simulink model "Vicon_server_multi_robot_test_3_robots"  (R2022b)
settings: Solver=ode2  StartTime=0.0  StopTime=inf  FixedStep=0.001  RelTol=1e-3  EnableMultiTasking=on
InitFcn:
  | %set_param('MS_FR/MISSION SERVER QDRONE POSITION CONTROL/Trajectory Enable', 'sw', '0' )
  | %set_param('MS_FR/MISSION SERVER QDRONE POSITION CONTROL/Command Enable', 'sw', '0' )
undefined symbols (not defined in the file or in its folder): qc_get_step_size
libraries: quarc_library x10, simulink x3
settings Model: SimulationMode=external  ExtModeTrigDuration=10000  Creator=Admin  LastModifiedBy=user
settings SolverCC: AlgebraicLoopSolver=TrustRegion  PositivePriorityOrder=on  AutoInsertRateTranBlk=on
settings DataIOCC: ReturnWorkspaceOutputs=off
settings DebuggingCC: UnconnectedInputMsg=warning  UnconnectedOutputMsg=warning  UnconnectedLineMsg=warning  SFUnexpectedBacktrackingDiag=warning  SFNoUnconditionalDefaultTransitionDiag=warning  SFExecutionAtInitializationDiag=none  SFMachineParentedDataDiag=warning  ArithmeticOperatorsInVariantConditions=warning
settings ModelReferenceCC: EnableRefExpFcnMdlSchedulingChecks=on
settings SFSimCC: SimUseLocalCustomCode=off  CustomCodeUndefinedFunction=UseInterfaceOnly
settings RTWCC: Description=QUARC Win64 Target Using Toolchain  SystemTargetFile=quarc_win64.tlc  TemplateMakefile=quarc_default_tmf  RTWUseLocalCustomCode=off  Toolchain=QUARC win64 | nmake (64-bit Windows)  BuildConfiguration=Faster Runs
settings CodeAppCC: StateflowObjectComments=on
settings STFCustomTargetCC: ConcurrentExecutionCompliant=on  GRTInterface=on  UseToolchainInfoCompliant=on  SystemTargetFile=quarc_win64.tlc
settings GRTTargetCC: TargetLangStandard=C89/C90 (ANSI)  ParMdlRefBuildCompliant=off  CompOptLevelCompliant=off  CombineOutputUpdateFcns=off  MatFileLogging=off  CPPClassGenCompliant=off  GRTInterface=on  ExtMode=on  ExtModeMexFile=quarc_comm  ExtModeMexArgs='-w -d %d -uri %u', 'tcpip://192.168.0.5:17005'
settings ConfigComp: CovMetricSettings=dw  CovSaveCumulativeToWorkspaceVar=on  CovSaveSingleToWorkspaceVar=on  CovExternalEMLEnable=off

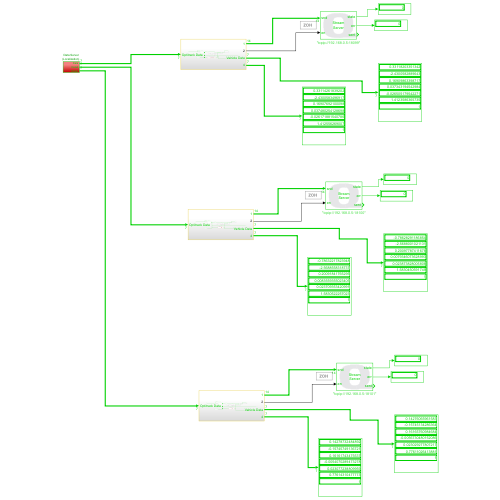
[thumbnail: Simulink's stored preview of the top-level diagram]
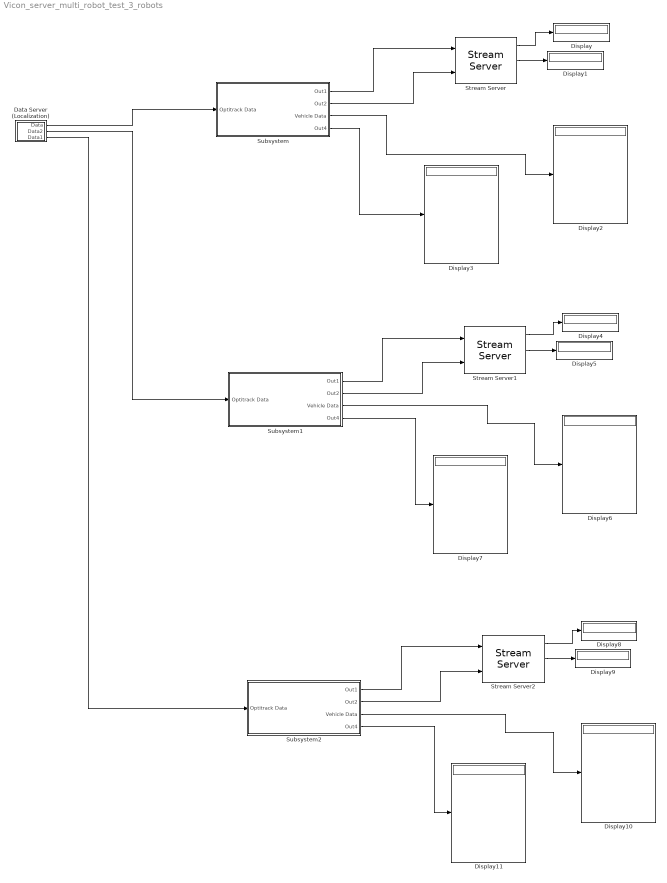
== system Vicon_server_multi_robot_test_3_robots ==
  "Data Server (Localization) " : Subsystem
  Display{,1..11} (12 alike) : Display
  Stream Server : quarc_library/Communications/Basic/Stream Server  uri_source=Specify via dialog (do not evaluate)  uri=tcpip://192.168.0.5:18099  send_buffer_size=1460  receive_buffer_size=1460  byte_order=little endian (Intel - LSB first)  optimization=Minimum latency  send_options=Send most recent data  receive_options=Do not receive data  default_value=[0]  sample_time=qc_get_step_size*2  active=off  implementation=Use blocking I/O in a separate thread  send_fifo_size=1000  receive_fifo_size=1000  send_priority=0  receive_priority=0  send_dimensions=off  receive_dimensions=off  max_dimensions=-1  data_type=Inherited via back propagation  type_expr=BusObject
      settings: AttributesFormatString="\"tcpip://192.168.0.5:18099\""
  Stream Server1 : quarc_library/Communications/Basic/Stream Server  uri_source=Specify via dialog (do not evaluate)  uri=tcpip://192.168.0.5:18100  send_buffer_size=1460  receive_buffer_size=1460  byte_order=little endian (Intel - LSB first)  optimization=Minimum latency  send_options=Send most recent data  receive_options=Do not receive data  default_value=[0]  sample_time=qc_get_step_size*2  active=off  implementation=Use blocking I/O in a separate thread  send_fifo_size=1000  receive_fifo_size=1000  send_priority=0  receive_priority=0  send_dimensions=off  receive_dimensions=off  max_dimensions=-1  data_type=Inherited via back propagation  type_expr=BusObject
      settings: AttributesFormatString="\"tcpip://192.168.0.5:18100\""
  Stream Server2 : quarc_library/Communications/Basic/Stream Server  uri_source=Specify via dialog (do not evaluate)  uri=tcpip://192.168.0.5:18101  send_buffer_size=1460  receive_buffer_size=1460  byte_order=little endian (Intel - LSB first)  optimization=Minimum latency  send_options=Send most recent data  receive_options=Do not receive data  default_value=[0]  sample_time=qc_get_step_size*2  active=off  implementation=Use blocking I/O in a separate thread  send_fifo_size=1000  receive_fifo_size=1000  send_priority=0  receive_priority=0  send_dimensions=off  receive_dimensions=off  max_dimensions=-1  data_type=Inherited via back propagation  type_expr=BusObject
      settings: AttributesFormatString="\"tcpip://192.168.0.5:18101\""
  Subsystem : Subsystem
  Subsystem1 : Subsystem
  Subsystem2 : Subsystem
  wires:
  Stream Server/1 -> Display/1
  Stream Server/2 -> Display1/1
  Subsystem/1(Out1) -> Stream Server/1
  Subsystem/2(Out2) -> Stream Server/2
  Subsystem/3(Vehicle Data) -> Display2/1
  Subsystem/4(Out4) -> Display3/1
  Stream Server1/1 -> Display4/1
  Stream Server1/2 -> Display5/1
  Subsystem1/4(Out4) -> Display7/1
  Subsystem1/1(Out1) -> Stream Server1/1
  Subsystem1/2(Out2) -> Stream Server1/2
  Subsystem1/3(Vehicle Data) -> Display6/1
  "Data Server (Localization) "/1(Data) -> Subsystem/1(Optitrack Data)
  "Data Server (Localization) "/2(Data2) -> Subsystem1/1(Optitrack Data)
  Subsystem2/2(Out2) -> Stream Server2/2
  Subsystem2/3(Vehicle Data) -> Display10/1
  Stream Server2/2 -> Display9/1
  Subsystem2/4(Out4) -> Display11/1
  Stream Server2/1 -> Display8/1
  Subsystem2/1(Out1) -> Stream Server2/1
  "Data Server (Localization) "/3(Data1) -> Subsystem2/1(Optitrack Data)

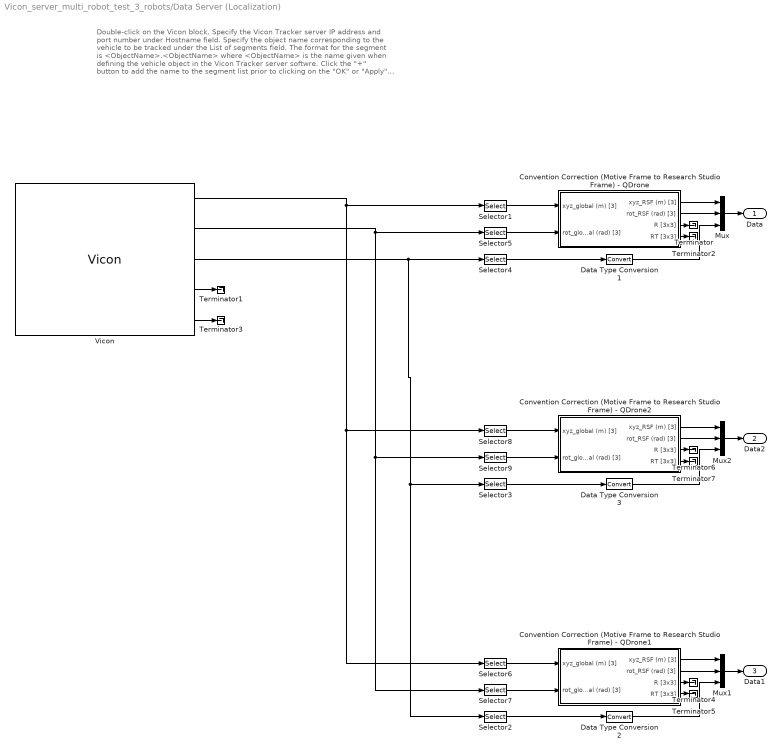
== system Vicon_server_multi_robot_test_3_robots/Data Server (Localization)  ==
  note: Double-click on the Vicon block.
      |
      | Specify the Vicon Tracker server IP address and port number under Hostname field.
      |
      | Specify the object name corresponding to the vehicle to be tracked under the
      | List of segments field. The format for the segment is <ObjectName>.<ObjectName>
      | where <ObjectName> is the name given when defining the vehicle object in the
      | Vicon Tracker server softwre. Click the "+" button to add the name to the segment list
      | prior to clicking on the "OK" or "Apply" button.
      | Remove extra/unused entries from the list using the "-" button.
      |
      | Make sure the checkbox next to the Object name inside the Object tab
      | in Vicon Tracker software is selected/checked and Tracker is streaming (Live) tracking
      | data before running this model.
  Convention Correction (Motive Frame to Research Studio Frame) - QDrone : Subsystem
  Convention Correction (Motive Frame to Research Studio Frame) - QDrone1 : Subsystem
  Convention Correction (Motive Frame to Research Studio Frame) - QDrone2 : Subsystem
  Data Type Conversion1 : DataTypeConversion  SaturateOnIntegerOverflow=off  RndMeth=Floor
  Data Type Conversion2 : DataTypeConversion  SaturateOnIntegerOverflow=off  RndMeth=Floor
  Data Type Conversion3 : DataTypeConversion  SaturateOnIntegerOverflow=off  RndMeth=Floor
  Mux : Mux  Inputs=3
  Mux1 : Mux  Inputs=3
  Mux2 : Mux  Inputs=3
  Selector1 : Selector  InputPortWidth=9  IndexOptions=Index vector (dialog)  Indices=[1:3]  OutputSizes=1
  Selector2 : Selector  InputPortWidth=3  IndexOptions=Index vector (dialog)  Indices=[3]  OutputSizes=1
  Selector3 : Selector  InputPortWidth=3  IndexOptions=Index vector (dialog)  Indices=[2]  OutputSizes=1
  Selector4 : Selector  InputPortWidth=3  IndexOptions=Index vector (dialog)  Indices=[1]  OutputSizes=1
  Selector5 : Selector  InputPortWidth=9  IndexOptions=Index vector (dialog)  Indices=[1:3]  OutputSizes=1
  Selector6 : Selector  InputPortWidth=9  IndexOptions=Index vector (dialog)  Indices=[7:9]  OutputSizes=1
  Selector7 : Selector  InputPortWidth=9  IndexOptions=Index vector (dialog)  Indices=[7:9]  OutputSizes=1
  Selector8 : Selector  InputPortWidth=9  IndexOptions=Index vector (dialog)  Indices=[4:6]  OutputSizes=1
  Selector9 : Selector  InputPortWidth=9  IndexOptions=Index vector (dialog)  Indices=[4:6]  OutputSizes=1
  Terminator{,1..7} (8 alike) : Terminator
  Vicon : quarc_library/Devices/Third-Party/Vicon/Vicon  hostname=192.168.10.1:801  segment_list=QBOT1.QBOT1\0QBOT2.QBOT2\0QBOT3.QBOT3\0\0  marker_list=\0  unlabeled_markers=[]  stream_mode=2  sample_time=qc_get_step_size*2  num_segments=3  num_markers=0  active=on
      settings: SourceProductName=QUARC Targets
  Data : Outport  VectorParamsAs1DForOutWhenUnconnected=off
  Data2 : Outport  Port=2  VectorParamsAs1DForOutWhenUnconnected=off
  Data1 : Outport  Port=3  VectorParamsAs1DForOutWhenUnconnected=off
  wires:
  Vicon/4 -> Terminator1/1
  Vicon/5 -> Terminator3/1
  Convention Correction (Motive Frame to Research Studio Frame) - QDrone/1(xyz_RSF (m) [3]) -> Mux/1
  Mux/1 -> Data/1
  Convention Correction (Motive Frame to Research Studio Frame) - QDrone/2(rot_RSF (rad) [3]) -> Mux/2
  Convention Correction (Motive Frame to Research Studio Frame) - QDrone/3(R [3x3]) -> Terminator/1
  Data Type Conversion1/1 -> Mux/3
  Convention Correction (Motive Frame to Research Studio Frame) - QDrone/4(RT [3x3]) -> Terminator2/1
  Convention Correction (Motive Frame to Research Studio Frame) - QDrone2/4(RT [3x3]) -> Terminator7/1
  Convention Correction (Motive Frame to Research Studio Frame) - QDrone2/1(xyz_RSF (m) [3]) -> Mux2/1
  Convention Correction (Motive Frame to Research Studio Frame) - QDrone2/2(rot_RSF (rad) [3]) -> Mux2/2
  Mux2/1 -> Data2/1
  Convention Correction (Motive Frame to Research Studio Frame) - QDrone2/3(R [3x3]) -> Terminator6/1
  Data Type Conversion3/1 -> Mux2/3
  Selector4/1 -> Data Type Conversion1/1
  Selector3/1 -> Data Type Conversion3/1
  Selector1/1 -> Convention Correction (Motive Frame to Research Studio Frame) - QDrone/1(xyz_global (m) [3])
  Selector5/1 -> Convention Correction (Motive Frame to Research Studio Frame) - QDrone/2(rot_global (rad) [3])
  Selector8/1 -> Convention Correction (Motive Frame to Research Studio Frame) - QDrone2/1(xyz_global (m) [3])
  Selector9/1 -> Convention Correction (Motive Frame to Research Studio Frame) - QDrone2/2(rot_global (rad) [3])
  Selector7/1 -> Convention Correction (Motive Frame to Research Studio Frame) - QDrone1/2(rot_global (rad) [3])
  Vicon/2 -> Selector7/1, Selector9/1, Selector5/1
  Convention Correction (Motive Frame to Research Studio Frame) - QDrone1/1(xyz_RSF (m) [3]) -> Mux1/1
  Selector6/1 -> Convention Correction (Motive Frame to Research Studio Frame) - QDrone1/1(xyz_global (m) [3])
  Data Type Conversion2/1 -> Mux1/3
  Vicon/3 -> Selector2/1, Selector3/1, Selector4/1
  Vicon/1 -> Selector6/1, Selector8/1, Selector1/1
  Selector2/1 -> Data Type Conversion2/1
  Convention Correction (Motive Frame to Research Studio Frame) - QDrone1/2(rot_RSF (rad) [3]) -> Mux1/2
  Mux1/1 -> Data1/1
  Convention Correction (Motive Frame to Research Studio Frame) - QDrone1/3(R [3x3]) -> Terminator4/1
  Convention Correction (Motive Frame to Research Studio Frame) - QDrone1/4(RT [3x3]) -> Terminator5/1

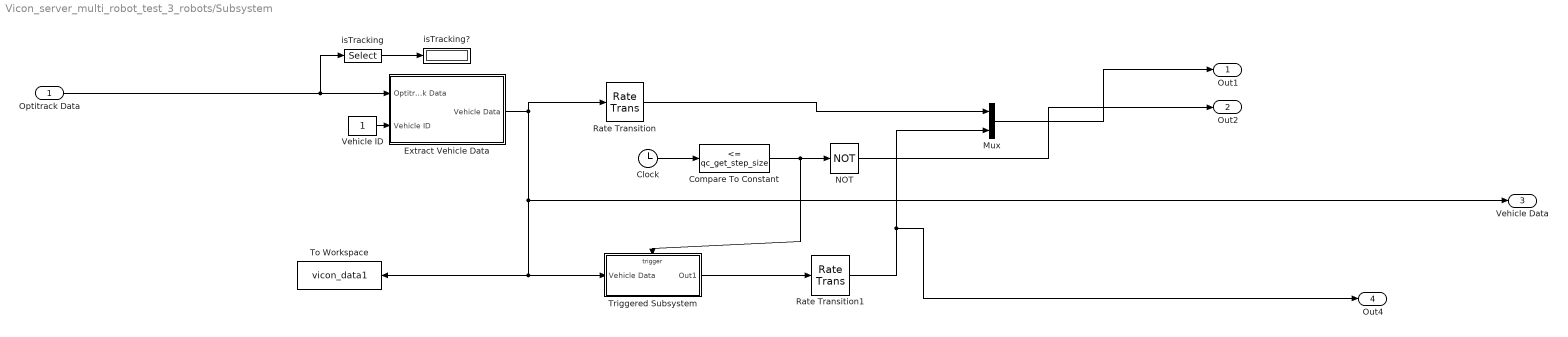
== system Vicon_server_multi_robot_test_3_robots/Subsystem ==
  Optitrack Data : Inport
  Clock : Clock
  Compare To Constant : simulink/Logic and Bit Operations/Compare To Constant  relop=<=  const=qc_get_step_size  OutDataTypeStr=boolean
  Extract Vehicle Data : Subsystem
  Mux : Mux  Inputs=2
  NOT : Logic  Operator=NOT  IconShape=distinctive  AllPortsSameDT=off  OutDataTypeStr=boolean
  Rate Transition : RateTransition  OutPortSampleTime=qc_get_step_size*2
  Rate Transition1 : RateTransition  OutPortSampleTime=qc_get_step_size*2
  To Workspace : ToWorkspace  VariableName=vicon_data1  SaveFormat=Structure With Time  SampleTime=-1
  Triggered Subsystem : Subsystem  TreatAsAtomicUnit=on
  Vehicle ID : Constant
  isTracking : Selector  InputPortWidth=7  IndexOptions=Index vector (dialog)  Indices=[7]  OutputSizes=1
  isTracking? : Display
  Out1 : Outport
  Out2 : Outport  Port=2
  Vehicle Data : Outport  Port=3
  Out4 : Outport  Port=4
  wires:
  Extract Vehicle Data/1(Vehicle Data) -> Vehicle Data/1, To Workspace/1, Triggered Subsystem/1(Vehicle Data), Rate Transition/1
  isTracking/1 -> isTracking?/1
  Compare To Constant/1 -> NOT/1, Triggered Subsystem/Trigger
  Vehicle ID/1 -> Extract Vehicle Data/2(Vehicle ID)
  Clock/1 -> Compare To Constant/1
  Rate Transition/1 -> Mux/1
  Triggered Subsystem/1(Out1) -> Rate Transition1/1
  Optitrack Data/1 -> Extract Vehicle Data/1(Optitrack Data), isTracking/1
  NOT/1 -> Out2/1
  Mux/1 -> Out1/1
  Rate Transition1/1 -> Out4/1, Mux/2

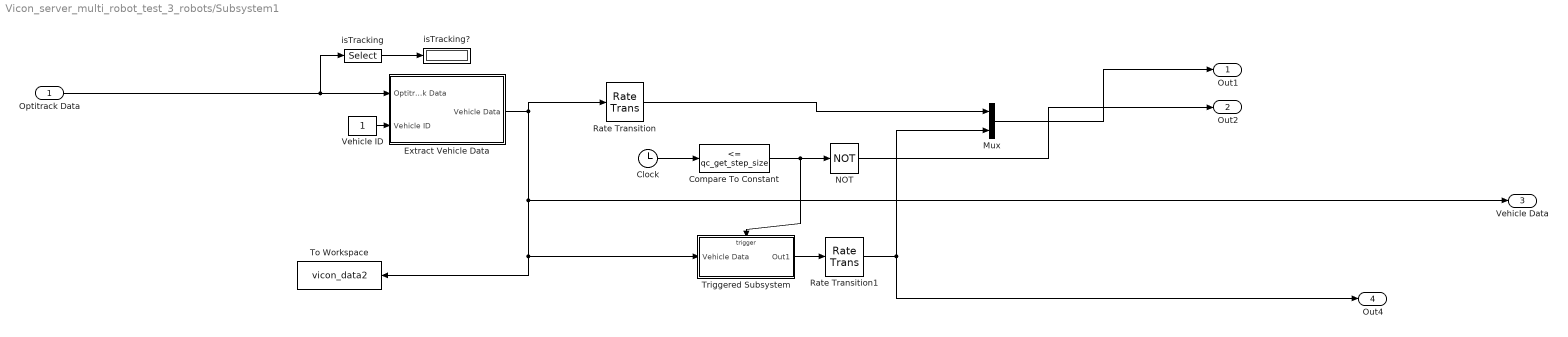
== system Vicon_server_multi_robot_test_3_robots/Subsystem1 ==
  Optitrack Data : Inport
  Clock : Clock
  Compare To Constant : simulink/Logic and Bit Operations/Compare To Constant  relop=<=  const=qc_get_step_size  OutDataTypeStr=boolean
  Extract Vehicle Data : Subsystem
  Mux : Mux  Inputs=2
  NOT : Logic  Operator=NOT  IconShape=distinctive  AllPortsSameDT=off  OutDataTypeStr=boolean
  Rate Transition : RateTransition  OutPortSampleTime=qc_get_step_size*2
  Rate Transition1 : RateTransition  OutPortSampleTime=qc_get_step_size*2
  To Workspace : ToWorkspace  VariableName=vicon_data2  SaveFormat=Structure With Time  SampleTime=-1
  Triggered Subsystem : Subsystem  TreatAsAtomicUnit=on
  Vehicle ID : Constant
  isTracking : Selector  InputPortWidth=7  IndexOptions=Index vector (dialog)  Indices=[7]  OutputSizes=1
  isTracking? : Display
  Out1 : Outport
  Out2 : Outport  Port=2
  Vehicle Data : Outport  Port=3
  Out4 : Outport  Port=4
  wires:
  Extract Vehicle Data/1(Vehicle Data) -> Vehicle Data/1, To Workspace/1, Triggered Subsystem/1(Vehicle Data), Rate Transition/1
  isTracking/1 -> isTracking?/1
  Compare To Constant/1 -> NOT/1, Triggered Subsystem/Trigger
  Vehicle ID/1 -> Extract Vehicle Data/2(Vehicle ID)
  Clock/1 -> Compare To Constant/1
  Rate Transition/1 -> Mux/1
  Triggered Subsystem/1(Out1) -> Rate Transition1/1
  Optitrack Data/1 -> Extract Vehicle Data/1(Optitrack Data), isTracking/1
  NOT/1 -> Out2/1
  Mux/1 -> Out1/1
  Rate Transition1/1 -> Mux/2, Out4/1

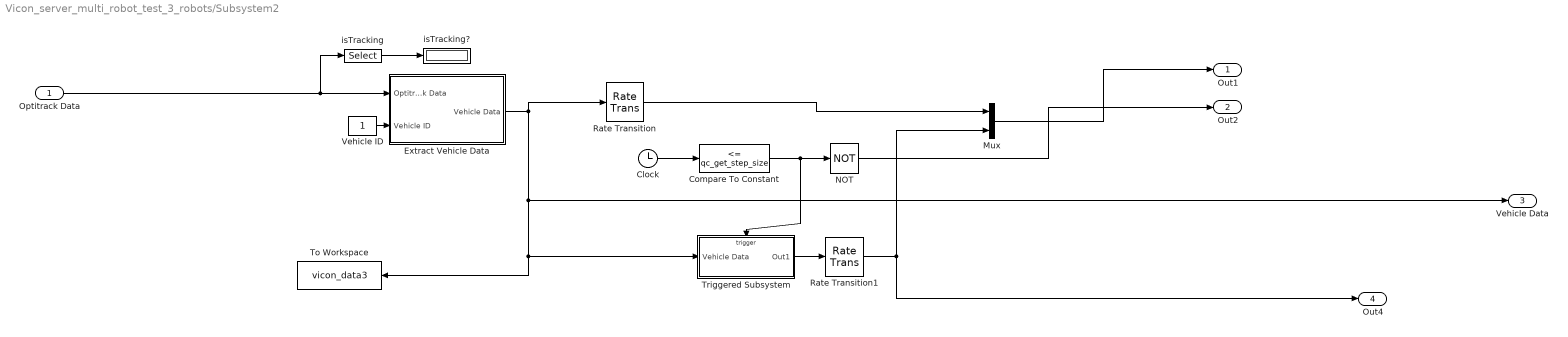
== system Vicon_server_multi_robot_test_3_robots/Subsystem2 ==
  Optitrack Data : Inport
  Clock : Clock
  Compare To Constant : simulink/Logic and Bit Operations/Compare To Constant  relop=<=  const=qc_get_step_size  OutDataTypeStr=boolean
  Extract Vehicle Data : Subsystem
  Mux : Mux  Inputs=2
  NOT : Logic  Operator=NOT  IconShape=distinctive  AllPortsSameDT=off  OutDataTypeStr=boolean
  Rate Transition : RateTransition  OutPortSampleTime=qc_get_step_size*2
  Rate Transition1 : RateTransition  OutPortSampleTime=qc_get_step_size*2
  To Workspace : ToWorkspace  VariableName=vicon_data3  SaveFormat=Structure With Time  SampleTime=-1
  Triggered Subsystem : Subsystem  TreatAsAtomicUnit=on
  Vehicle ID : Constant
  isTracking : Selector  InputPortWidth=7  IndexOptions=Index vector (dialog)  Indices=[7]  OutputSizes=1
  isTracking? : Display
  Out1 : Outport
  Out2 : Outport  Port=2
  Vehicle Data : Outport  Port=3
  Out4 : Outport  Port=4
  wires:
  Extract Vehicle Data/1(Vehicle Data) -> Vehicle Data/1, To Workspace/1, Triggered Subsystem/1(Vehicle Data), Rate Transition/1
  isTracking/1 -> isTracking?/1
  Compare To Constant/1 -> NOT/1, Triggered Subsystem/Trigger
  Vehicle ID/1 -> Extract Vehicle Data/2(Vehicle ID)
  Clock/1 -> Compare To Constant/1
  Rate Transition/1 -> Mux/1
  Triggered Subsystem/1(Out1) -> Rate Transition1/1
  Optitrack Data/1 -> Extract Vehicle Data/1(Optitrack Data), isTracking/1
  NOT/1 -> Out2/1
  Mux/1 -> Out1/1
  Rate Transition1/1 -> Mux/2, Out4/1

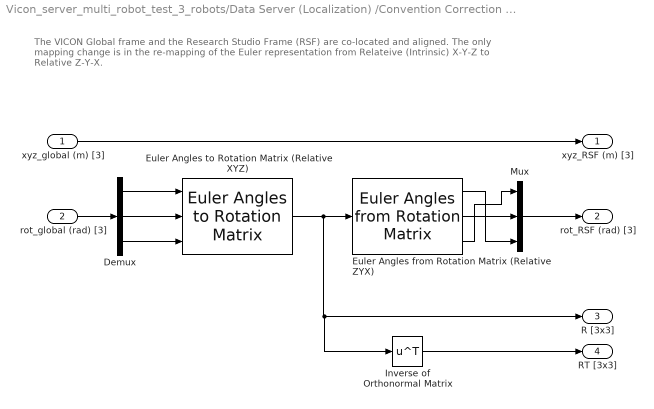
== system Vicon_server_multi_robot_test_3_robots/Data Server (Localization) /Convention Correction (Motive Frame to Research Studio Frame) - QDrone ==
  note: The VICON Global frame and the Research Studio Frame (RSF) are co-located and aligned.
      | The only mapping change is in the re-mapping of the Euler representation from
      | Relateive (Intrinsic) X-Y-Z to Relative Z-Y-X.
  xyz_global (m) [3] : Inport
  rot_global (rad) [3] : Inport  Port=2
  Demux : Demux  Outputs=3
  Euler Angles from Rotation Matrix (Relative ZYX) : quarc_library/Math Operations/Matrices/Euler Angles from Rotation Matrix  menu_order=Relative Z-Y-X
      settings: SourceProductName=QUARC Targets
  Euler Angles to Rotation Matrix (Relative XYZ) : quarc_library/Math Operations/Matrices/Euler Angles to Rotation Matrix  menu_order=Relative X-Y-Z
      settings: SourceProductName=QUARC Targets
  Inverse of Orthonormal Matrix : Math  Operator=transpose  SignedPower=on
  Mux : Mux  Inputs=3
  xyz_RSF (m) [3] : Outport  VectorParamsAs1DForOutWhenUnconnected=off
  rot_RSF (rad) [3] : Outport  Port=2  VectorParamsAs1DForOutWhenUnconnected=off
  R [3x3] : Outport  Port=3  VectorParamsAs1DForOutWhenUnconnected=off
  RT [3x3] : Outport  Port=4  VectorParamsAs1DForOutWhenUnconnected=off
  wires:
  Inverse of Orthonormal Matrix/1 -> RT [3x3]/1
  Euler Angles to Rotation Matrix (Relative XYZ)/1 -> Euler Angles from Rotation Matrix (Relative ZYX)/1, R [3x3]/1, Inverse of Orthonormal Matrix/1
  Euler Angles from Rotation Matrix (Relative ZYX)/2 -> Mux/2
  Euler Angles from Rotation Matrix (Relative ZYX)/3 -> Mux/1
  Mux/1 -> rot_RSF (rad) [3]/1
  Euler Angles from Rotation Matrix (Relative ZYX)/1 -> Mux/3
  xyz_global (m) [3]/1 -> xyz_RSF (m) [3]/1
  Demux/2 -> Euler Angles to Rotation Matrix (Relative XYZ)/2
  rot_global (rad) [3]/1 -> Demux/1
  Demux/1 -> Euler Angles to Rotation Matrix (Relative XYZ)/1
  Demux/3 -> Euler Angles to Rotation Matrix (Relative XYZ)/3

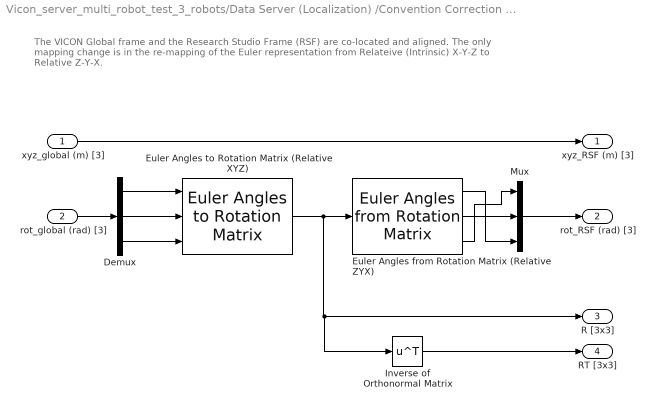
== system Vicon_server_multi_robot_test_3_robots/Data Server (Localization) /Convention Correction (Motive Frame to Research Studio Frame) - QDrone1 ==
  note: The VICON Global frame and the Research Studio Frame (RSF) are co-located and aligned.
      | The only mapping change is in the re-mapping of the Euler representation from
      | Relateive (Intrinsic) X-Y-Z to Relative Z-Y-X.
  xyz_global (m) [3] : Inport
  rot_global (rad) [3] : Inport  Port=2
  Demux : Demux  Outputs=3
  Euler Angles from Rotation Matrix (Relative ZYX) : quarc_library/Math Operations/Matrices/Euler Angles from Rotation Matrix  menu_order=Relative Z-Y-X
      settings: SourceProductName=QUARC Targets
  Euler Angles to Rotation Matrix (Relative XYZ) : quarc_library/Math Operations/Matrices/Euler Angles to Rotation Matrix  menu_order=Relative X-Y-Z
      settings: SourceProductName=QUARC Targets
  Inverse of Orthonormal Matrix : Math  Operator=transpose  SignedPower=on
  Mux : Mux  Inputs=3
  xyz_RSF (m) [3] : Outport  VectorParamsAs1DForOutWhenUnconnected=off
  rot_RSF (rad) [3] : Outport  Port=2  VectorParamsAs1DForOutWhenUnconnected=off
  R [3x3] : Outport  Port=3  VectorParamsAs1DForOutWhenUnconnected=off
  RT [3x3] : Outport  Port=4  VectorParamsAs1DForOutWhenUnconnected=off
  wires:
  Inverse of Orthonormal Matrix/1 -> RT [3x3]/1
  Euler Angles to Rotation Matrix (Relative XYZ)/1 -> Euler Angles from Rotation Matrix (Relative ZYX)/1, R [3x3]/1, Inverse of Orthonormal Matrix/1
  Euler Angles from Rotation Matrix (Relative ZYX)/2 -> Mux/2
  Euler Angles from Rotation Matrix (Relative ZYX)/3 -> Mux/1
  Mux/1 -> rot_RSF (rad) [3]/1
  Euler Angles from Rotation Matrix (Relative ZYX)/1 -> Mux/3
  xyz_global (m) [3]/1 -> xyz_RSF (m) [3]/1
  Demux/2 -> Euler Angles to Rotation Matrix (Relative XYZ)/2
  rot_global (rad) [3]/1 -> Demux/1
  Demux/1 -> Euler Angles to Rotation Matrix (Relative XYZ)/1
  Demux/3 -> Euler Angles to Rotation Matrix (Relative XYZ)/3

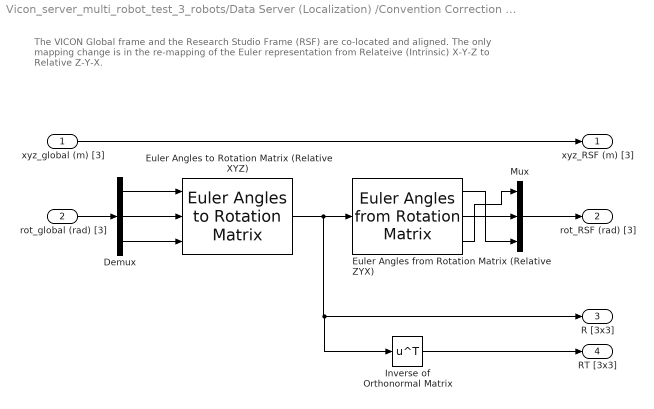
== system Vicon_server_multi_robot_test_3_robots/Data Server (Localization) /Convention Correction (Motive Frame to Research Studio Frame) - QDrone2 ==
  note: The VICON Global frame and the Research Studio Frame (RSF) are co-located and aligned.
      | The only mapping change is in the re-mapping of the Euler representation from
      | Relateive (Intrinsic) X-Y-Z to Relative Z-Y-X.
  xyz_global (m) [3] : Inport
  rot_global (rad) [3] : Inport  Port=2
  Demux : Demux  Outputs=3
  Euler Angles from Rotation Matrix (Relative ZYX) : quarc_library/Math Operations/Matrices/Euler Angles from Rotation Matrix  menu_order=Relative Z-Y-X
      settings: SourceProductName=QUARC Targets
  Euler Angles to Rotation Matrix (Relative XYZ) : quarc_library/Math Operations/Matrices/Euler Angles to Rotation Matrix  menu_order=Relative X-Y-Z
      settings: SourceProductName=QUARC Targets
  Inverse of Orthonormal Matrix : Math  Operator=transpose  SignedPower=on
  Mux : Mux  Inputs=3
  xyz_RSF (m) [3] : Outport  VectorParamsAs1DForOutWhenUnconnected=off
  rot_RSF (rad) [3] : Outport  Port=2  VectorParamsAs1DForOutWhenUnconnected=off
  R [3x3] : Outport  Port=3  VectorParamsAs1DForOutWhenUnconnected=off
  RT [3x3] : Outport  Port=4  VectorParamsAs1DForOutWhenUnconnected=off
  wires:
  Inverse of Orthonormal Matrix/1 -> RT [3x3]/1
  Euler Angles to Rotation Matrix (Relative XYZ)/1 -> Euler Angles from Rotation Matrix (Relative ZYX)/1, R [3x3]/1, Inverse of Orthonormal Matrix/1
  Euler Angles from Rotation Matrix (Relative ZYX)/2 -> Mux/2
  Euler Angles from Rotation Matrix (Relative ZYX)/3 -> Mux/1
  Mux/1 -> rot_RSF (rad) [3]/1
  Euler Angles from Rotation Matrix (Relative ZYX)/1 -> Mux/3
  xyz_global (m) [3]/1 -> xyz_RSF (m) [3]/1
  Demux/2 -> Euler Angles to Rotation Matrix (Relative XYZ)/2
  rot_global (rad) [3]/1 -> Demux/1
  Demux/1 -> Euler Angles to Rotation Matrix (Relative XYZ)/1
  Demux/3 -> Euler Angles to Rotation Matrix (Relative XYZ)/3

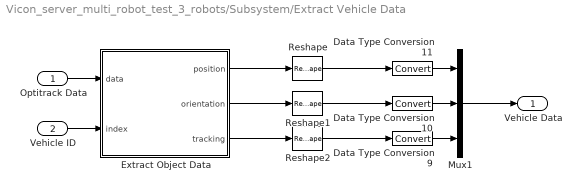
== system Vicon_server_multi_robot_test_3_robots/Subsystem/Extract Vehicle Data ==
  Optitrack Data : Inport
  Vehicle ID : Inport  Port=2
  Data Type Conversion10 : DataTypeConversion  SaturateOnIntegerOverflow=off  RndMeth=Floor
  Data Type Conversion11 : DataTypeConversion  SaturateOnIntegerOverflow=off  RndMeth=Floor
  Data Type Conversion9 : DataTypeConversion  SaturateOnIntegerOverflow=off  RndMeth=Floor
  Extract Object Data : MATLAB Function  TreatAsAtomicUnit=on
  Mux1 : Mux  Inputs=3
  Reshape : Reshape
  Reshape1 : Reshape
  Reshape2 : Reshape
  Vehicle Data : Outport  VectorParamsAs1DForOutWhenUnconnected=off
  wires:
  Vehicle ID/1 -> Extract Object Data/2(index)
  Optitrack Data/1 -> Extract Object Data/1(data)
  Mux1/1 -> Vehicle Data/1
  Extract Object Data/1(position) -> Reshape/1
  Extract Object Data/3(tracking) -> Reshape2/1
  Extract Object Data/2(orientation) -> Reshape1/1
  Data Type Conversion11/1 -> Mux1/1
  Data Type Conversion10/1 -> Mux1/2
  Data Type Conversion9/1 -> Mux1/3
  Reshape/1 -> Data Type Conversion11/1
  Reshape1/1 -> Data Type Conversion10/1
  Reshape2/1 -> Data Type Conversion9/1

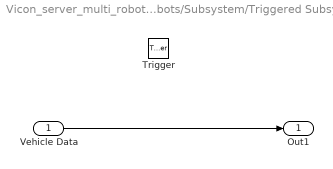
== system Vicon_server_multi_robot_test_3_robots/Subsystem/Triggered Subsystem ==
  Vehicle Data : Inport
  Trigger : TriggerPort  TriggerType=falling  VariantControl=(inherit)
  Out1 : Outport
  wires:
  Vehicle Data/1 -> Out1/1

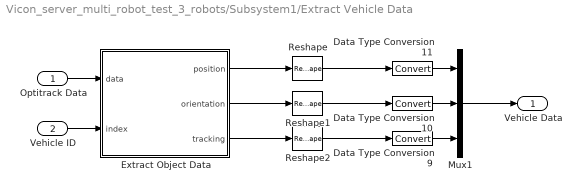
== system Vicon_server_multi_robot_test_3_robots/Subsystem1/Extract Vehicle Data ==
  Optitrack Data : Inport
  Vehicle ID : Inport  Port=2
  Data Type Conversion10 : DataTypeConversion  SaturateOnIntegerOverflow=off  RndMeth=Floor
  Data Type Conversion11 : DataTypeConversion  SaturateOnIntegerOverflow=off  RndMeth=Floor
  Data Type Conversion9 : DataTypeConversion  SaturateOnIntegerOverflow=off  RndMeth=Floor
  Extract Object Data : MATLAB Function  TreatAsAtomicUnit=on
  Mux1 : Mux  Inputs=3
  Reshape : Reshape
  Reshape1 : Reshape
  Reshape2 : Reshape
  Vehicle Data : Outport  VectorParamsAs1DForOutWhenUnconnected=off
  wires:
  Vehicle ID/1 -> Extract Object Data/2(index)
  Optitrack Data/1 -> Extract Object Data/1(data)
  Mux1/1 -> Vehicle Data/1
  Extract Object Data/1(position) -> Reshape/1
  Extract Object Data/3(tracking) -> Reshape2/1
  Extract Object Data/2(orientation) -> Reshape1/1
  Data Type Conversion11/1 -> Mux1/1
  Data Type Conversion10/1 -> Mux1/2
  Data Type Conversion9/1 -> Mux1/3
  Reshape/1 -> Data Type Conversion11/1
  Reshape1/1 -> Data Type Conversion10/1
  Reshape2/1 -> Data Type Conversion9/1

== system Vicon_server_multi_robot_test_3_robots/Subsystem1/Triggered Subsystem ==
  Vehicle Data : Inport
  Trigger : TriggerPort  TriggerType=falling  VariantControl=(inherit)
  Out1 : Outport
  wires:
  Vehicle Data/1 -> Out1/1

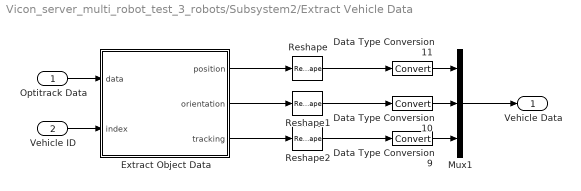
== system Vicon_server_multi_robot_test_3_robots/Subsystem2/Extract Vehicle Data ==
  Optitrack Data : Inport
  Vehicle ID : Inport  Port=2
  Data Type Conversion10 : DataTypeConversion  SaturateOnIntegerOverflow=off  RndMeth=Floor
  Data Type Conversion11 : DataTypeConversion  SaturateOnIntegerOverflow=off  RndMeth=Floor
  Data Type Conversion9 : DataTypeConversion  SaturateOnIntegerOverflow=off  RndMeth=Floor
  Extract Object Data : MATLAB Function  TreatAsAtomicUnit=on
  Mux1 : Mux  Inputs=3
  Reshape : Reshape
  Reshape1 : Reshape
  Reshape2 : Reshape
  Vehicle Data : Outport  VectorParamsAs1DForOutWhenUnconnected=off
  wires:
  Vehicle ID/1 -> Extract Object Data/2(index)
  Optitrack Data/1 -> Extract Object Data/1(data)
  Mux1/1 -> Vehicle Data/1
  Extract Object Data/1(position) -> Reshape/1
  Extract Object Data/3(tracking) -> Reshape2/1
  Extract Object Data/2(orientation) -> Reshape1/1
  Data Type Conversion11/1 -> Mux1/1
  Data Type Conversion10/1 -> Mux1/2
  Data Type Conversion9/1 -> Mux1/3
  Reshape/1 -> Data Type Conversion11/1
  Reshape1/1 -> Data Type Conversion10/1
  Reshape2/1 -> Data Type Conversion9/1

== system Vicon_server_multi_robot_test_3_robots/Subsystem2/Triggered Subsystem ==
  Vehicle Data : Inport
  Trigger : TriggerPort  TriggerType=falling  VariantControl=(inherit)
  Out1 : Outport
  wires:
  Vehicle Data/1 -> Out1/1

== matlab function Vicon_server_multi_robot_test_3_robots/Subsystem/Extract Vehicle Data/Extract Object Data ==
  data: data input; position output; orientation output; index input; tracking output
function [position, orientation, tracking] = fcn(data, index)

n = length(data)/7;

if (index<=0)||(index>n)
    position = zeros(1,3); orientation = zeros(1,3); tracking = 0;
else
    position = [data(index*3-2), data(index*3-1), data(index*3)];
    orientation = [data((index+n)*3 - 2), data((index+n)*3 - 1), data((index+n)*3)];
    tracking = data(index + (n*6));
end

== matlab function Vicon_server_multi_robot_test_3_robots/Subsystem1/Extract Vehicle Data/Extract Object Data ==
  data: data input; position output; orientation output; index input; tracking output
function [position, orientation, tracking] = fcn(data, index)

n = length(data)/7;

if (index<=0)||(index>n)
    position = zeros(1,3); orientation = zeros(1,3); tracking = 0;
else
    position = [data(index*3-2), data(index*3-1), data(index*3)];
    orientation = [data((index+n)*3 - 2), data((index+n)*3 - 1), data((index+n)*3)];
    tracking = data(index + (n*6));
end

== matlab function Vicon_server_multi_robot_test_3_robots/Subsystem2/Extract Vehicle Data/Extract Object Data ==
  data: data input; position output; orientation output; index input; tracking output
function [position, orientation, tracking] = fcn(data, index)

n = length(data)/7;

if (index<=0)||(index>n)
    position = zeros(1,3); orientation = zeros(1,3); tracking = 0;
else
    position = [data(index*3-2), data(index*3-1), data(index*3)];
    orientation = [data((index+n)*3 - 2), data((index+n)*3 - 1), data((index+n)*3)];
    tracking = data(index + (n*6));
end
